simulink model "verify_Roof_mdl"  (R2018b)
settings: Solver=ode45  StartTime=0  StopTime=24*3600  MaxStep=100  RelTol=1e-3  EnableMultiTasking=on
libraries: carnot x4
settings Model: Creator=drhf  LastModifiedBy=drhf
settings DataIOCC: SaveFormat=Array  SignalLoggingSaveFormat=ModelDataLogs
settings OptimizationCC: ExpressionDepthLimit=2147483647  LifeSpan=inf
settings DebuggingCC: UnderspecifiedInitializationDetection=Classic  MergeDetectMultiDrivingBlocksExec=none  SolverPrmCheckMsg=warning  FcnCallInpInsideContextMsg=warning  StateNameClashWarn=warning  SFUnexpectedBacktrackingDiag=warning  SFNoUnconditionalDefaultTransitionDiag=warning  SFExecutionAtInitializationDiag=none
settings HardwareCC: ProdBitPerPointer=32  ProdBitPerSizeT=32  ProdBitPerPtrDiffT=32  ProdLargestAtomicFloat=None  ProdIntDivRoundTo=Undefined  ProdEndianess=Unspecified  ProdWordSize=32  ProdHWDeviceType=32-bit Generic
settings ModelReferenceCC: PropagateSignalLabelsOutOfModel=off
settings SFSimCC: SimUseLocalCustomCode=off
settings RTWCC: RTWUseLocalCustomCode=off
settings CodeAppCC: StateflowObjectComments=on
settings GRTTargetCC: TargetLangStandard=C89/C90 (ANSI)  GeneratePreprocessorConditionals=Disable all  CombineOutputUpdateFcns=off  GRTInterface=on
settings ConfigComp: CovMetricSettings=dw  CovHtmlReporting=on  CovSaveCumulativeToWorkspaceVar=on  CovSaveSingleToWorkspaceVar=on  CovExternalEMLEnable=off

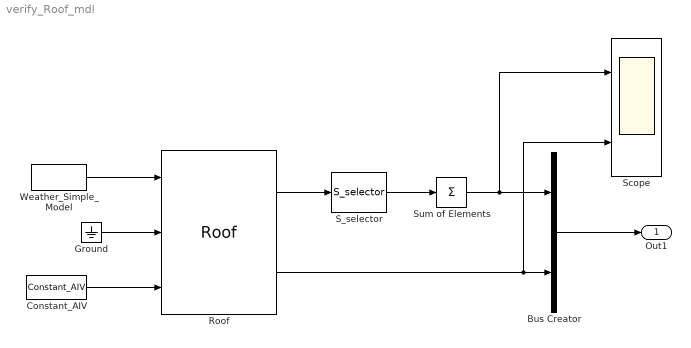
== system verify_Roof_mdl ==
  Bus Creator : BusCreator  Inputs=2
  Constant_AIV : carnot/Source/Ventilation/Constant_AIV  Tsens=20  Tcon=20  Trad=20  mw=0.012  mco=0.01  rhoair=1.2  cpair=1004  pair=100000  nair=0.5
  Ground : Ground
  Roof : carnot/Basic/Thermal_Models/Roof  wallsize=[5 5]  pos=[0 0 0]  t0=10  d=[0.015 0.38 0.02]  cond=[1.4 0.79 0.7]  cwall=[0.28 0.28 0.28]*3600  rho=[2000 1800 1400]  reflectground=0.2  abs_emiss=[0.6, 0.9, 0.9]  tau=10  dactive=-1
  S_selector : carnot/Outputs/S_selector  e1=off  e2=off  e3=off  e4=off  e5=off  e6=off  e7=on  e8=on  e9=off  e10=off  e11=off  e12=off  e13=off
  Scope : Scope  NumInputPorts=2
  Sum of Elements : Sum  Inputs=+
  Weather_Simple_Model : carnot/Weather/Weather_Simple_Model  lat=60  Ibn=900  Idg=100  tamb=5  deltaTsky=-6  rh=50  precip="10e-3/24/3600           % 10 mm in 24 h"  cloud=0.125  p=1013e2  vw=1  wdir=270
  Out1 : Outport
  wires:
  Bus Creator/1 -> Out1/1
  Roof/1 -> S_selector/1
  S_selector/1 -> Sum of Elements/1
  Sum of Elements/1 -> Scope/1, Bus Creator/1
  Ground/1 -> Roof/2
  Constant_AIV/1 -> Roof/3
  Roof/2 -> Scope/2, Bus Creator/2
  Weather_Simple_Model/1 -> Roof/1
